simulink model "SF009A_DutyCycThermProtn"  (R2013b)
settings: Solver=FixedStepDiscrete  SolverMode=SingleTasking  StartTime=0.0  StopTime=1  FixedStep=0.1  RelTol=1e-3
values from neighbouring files (symbols this model uses):
  AbsltTThermLimCnt = DataDict.NTC    [SF009A_DutyCycThermProtn_DataDict.m]
  ARCHGLBPRM_100MILLISEC_SEC_F32 = DataDict.Constant    [SF009A_DutyCycThermProtn_DataDict.m]
  CTRLRANDCUTFLT_CNT_U08 = DataDict.Constant    [SF009A_DutyCycThermProtn_DataDict.m]
  CTRLRTFLT_CNT_U08 = DataDict.Constant    [SF009A_DutyCycThermProtn_DataDict.m]
  CUTFLT_CNT_U08 = DataDict.Constant    [SF009A_DutyCycThermProtn_DataDict.m]
  DITHERMLIM_MOTNWTMTR_F32 = DataDict.Constant    [SF009A_DutyCycThermProtn_DataDict.m]
  DutyCycExcddCnt = DataDict.NTC    [SF009A_DutyCycThermProtn_DataDict.m]
  DutyCycThermProtnAbsltCtrlTTblX = DataDict.Calibration    [SF009A_DutyCycThermProtn_DataDict.m]
  DutyCycThermProtnAbsltCtrlTTqTblY = DataDict.Calibration    [SF009A_DutyCycThermProtn_DataDict.m]
  DutyCycThermProtnAbsltCuTTblX = DataDict.Calibration    [SF009A_DutyCycThermProtn_DataDict.m]
  DutyCycThermProtnAbsltCuTTqTblY = DataDict.Calibration    [SF009A_DutyCycThermProtn_DataDict.m]
  DutyCycThermProtnAbsltMotVelBreakPt = DataDict.Calibration    [SF009A_DutyCycThermProtn_DataDict.m]
  DutyCycThermProtnAbsltTTqSlewHiLim = DataDict.Calibration    [SF009A_DutyCycThermProtn_DataDict.m]
  DutyCycThermProtnAbsltTTqSlewLoLim = DataDict.Calibration    [SF009A_DutyCycThermProtn_DataDict.m]
  DutyCycThermProtnCtrlT = DataDict.Calibration    [SF009A_DutyCycThermProtn_DataDict.m]
  DutyCycThermProtnCtrlTSeln = DataDict.Calibration    [SF009A_DutyCycThermProtn_DataDict.m]
  DutyCycThermProtnDutyCycFildThd = DataDict.Calibration    [SF009A_DutyCycThermProtn_DataDict.m]
  DutyCycThermProtnIgnOffCtrlEna = DataDict.Calibration    [SF009A_DutyCycThermProtn_DataDict.m]
  DutyCycThermProtnIgnOffMsgWaitTi = DataDict.Calibration    [SF009A_DutyCycThermProtn_DataDict.m]
  DutyCycThermProtnLstTblValNonStall = DataDict.Calibration    [SF009A_DutyCycThermProtn_DataDict.m]
  DutyCycThermProtnLstTblValStall = DataDict.Calibration    [SF009A_DutyCycThermProtn_DataDict.m]
  DutyCycThermProtnMotPrTSeln = DataDict.Calibration    [SF009A_DutyCycThermProtn_DataDict.m]
  DutyCycThermProtnMplr1NonStallTblY = DataDict.Calibration    [SF009A_DutyCycThermProtn_DataDict.m]
  DutyCycThermProtnMplr1StallTblY = DataDict.Calibration    [SF009A_DutyCycThermProtn_DataDict.m]
  DutyCycThermProtnMplr2NonStallTblY = DataDict.Calibration    [SF009A_DutyCycThermProtn_DataDict.m]
  DutyCycThermProtnMplr2StallTblY = DataDict.Calibration    [SF009A_DutyCycThermProtn_DataDict.m]
  DutyCycThermProtnMplr3NonStallTblY = DataDict.Calibration    [SF009A_DutyCycThermProtn_DataDict.m]
  DutyCycThermProtnMplr3StallTblY = DataDict.Calibration    [SF009A_DutyCycThermProtn_DataDict.m]
  DutyCycThermProtnMplr4NonStallTblY = DataDict.Calibration    [SF009A_DutyCycThermProtn_DataDict.m]
  DutyCycThermProtnMplr4StallTblY = DataDict.Calibration    [SF009A_DutyCycThermProtn_DataDict.m]
  DutyCycThermProtnMplr5NonStallTblY = DataDict.Calibration    [SF009A_DutyCycThermProtn_DataDict.m]
  DutyCycThermProtnMplr5StallTblY = DataDict.Calibration    [SF009A_DutyCycThermProtn_DataDict.m]
  DutyCycThermProtnMplr6NonStallTblY = DataDict.Calibration    [SF009A_DutyCycThermProtn_DataDict.m]
  DutyCycThermProtnMplr6StallTblY = DataDict.Calibration    [SF009A_DutyCycThermProtn_DataDict.m]
  DutyCycThermProtnMplrTblX = DataDict.Calibration    [SF009A_DutyCycThermProtn_DataDict.m]
  DutyCycThermProtnMplrTSeln = DataDict.Calibration    [SF009A_DutyCycThermProtn_DataDict.m]
  DutyCycThermProtnSlowFilTSeln = DataDict.Calibration    [SF009A_DutyCycThermProtn_DataDict.m]
  DutyCycThermProtnThermLimScaFac = DataDict.Calibration    [SF009A_DutyCycThermProtn_DataDict.m]
  DutyCycThermProtnThermLoadLimTblX = DataDict.Calibration    [SF009A_DutyCycThermProtn_DataDict.m]
  DutyCycThermProtnThermLoadLimTblY = DataDict.Calibration    [SF009A_DutyCycThermProtn_DataDict.m]
  DutyCycThermProtnTqCmdSlewDwn = DataDict.Calibration    [SF009A_DutyCycThermProtn_DataDict.m]
  DutyCycThermProtnTqCmdSlewUp = DataDict.Calibration    [SF009A_DutyCycThermProtn_DataDict.m]
  FILVALMIN_ULS_F32 = DataDict.Constant    [SF009A_DutyCycThermProtn_DataDict.m]
  IGNTIOFFTHD_CNT_F32 = DataDict.Constant    [SF009A_DutyCycThermProtn_DataDict.m]
  NODEBSTEP_CNT_U16 = DataDict.Constant    [SF009A_DutyCycThermProtn_DataDict.m]
  ONEPERC_ULS_F32 = DataDict.Constant    [SF009A_DutyCycThermProtn_DataDict.m]
  TAU3_SEC_F32 = DataDict.Constant    [SF009A_DutyCycThermProtn_DataDict.m]
  TAU4_SEC_F32 = DataDict.Constant    [SF009A_DutyCycThermProtn_DataDict.m]
  TAU5_SEC_F32 = DataDict.Constant    [SF009A_DutyCycThermProtn_DataDict.m]
  TAU6_SEC_F32 = DataDict.Constant    [SF009A_DutyCycThermProtn_DataDict.m]
  THERMLOADLIMTBLIDX_ULS_U08 = DataDict.Constant    [SF009A_DutyCycThermProtn_DataDict.m]
undefined symbols (not defined in the file or in its folder): NtcSts1, NvmGetErrSts1
libraries: FixdToFloat x13, Fil x12, NxtrLim x12, simulink x11, NxtrMath x8, FloatToFixd x6, NxtrMax x6, NxtrMin x3, NxtrAbslt x2, NxtrNvM x1
(part 6 of 7)

== system SF009A_DutyCycThermProtn/DutyCycThermProtn/DutyCycThermProtnPer1/LoadLimiting/Multiplier/NonStallCondition ==
  note: Lookup table structure for all tables changed from interpolation to step change for each temperature range.
      | For input values less than the first calibrated X value, the first Y value shall be used, and for input values greater than the largest calibrated X value, the last Y value shall be used.
  note: Non-Stall Condition
  note: Lookup method : Use Input below
  note: Lookup method : Use Input below
  note: Lookup method : Use Input below
  note: Lookup method : Use Input below
  note: Lookup method : Use Input below
  note: Lookup method : Use Input below
  note: The Lookup method used for all the 6 tables below is  "Use Input below" meaning Finds the element in x nearest and below the current input.
      | The corresponding element in y is the output. If there is no element in x below thecurrent input, the block finds the nearest element.
  Mult12Temp : Inport  RequirementInfo={'linktype_rmi_doors' '0000a52a (/E-STEER Core/SubSystem Specifications/Application Functions/SF009A Thermal Duty Cycle Protection)' '#SF009A_224' 'true' 'REQ: SF009A_224' '' } %GIDa_15a3ec26_ae13_4a01_898e_d603e4d6290a
  Mult36TempSlc : Inport  RequirementInfo={'linktype_rmi_doors' '0000a52a (/E-STEER Core/SubSystem Specifications/Application Functions/SF009A Thermal Duty Cycle Protection)' '#SF009A_225' 'true' 'REQ: SF009A_225' '' } %GIDa_709b3fc5_f20d_404f_aaf0_efd71be834f5  Port=2
  Action Port : ActionPort  ActionType=then
  CopyRight2 : Subsystem  Description=|  mask(Copyright Information){none=on}
      | Copyright info block.                                               
      |                                                                     
      | Place copyright information at the top of every subsystem in design.
      mask prompts: none "No parameters"
      mask help: Place copyright information at the top of every subsystem in design.
      mask Display:
      | NxtrConf = 'Nexteer Confidential';
      | 
      | sys = bdroot; %handle for the current model ("system")
      | first = get_param(sys,'Created');
      | first = first(end-3:end);  %year is last four digits
      | 
      | last = get_param(sys,'LastModifiedDate');
      | if isempty(last)
      |     last = datestr(now,'yyyy');
      | else
      |     last = last(end-3:end);
      | end
      | 
      | if strcmp(first,last)
      |     fprintf('%s -- Copyright %s Nexteer',NxtrConf,first)
      | else
      |     fprintf('%s -- %s%s- %s Nexteer',NxtrConf,char(169),first,last)
      | end
  Multiplier 1 Non-Stall Condition Table Lookup : Lookup  RequirementInfo={'linktype_rmi_doors' '0000a52a (/E-STEER Core/SubSystem Specifications/Application Functions/SF009A Thermal Duty Cycle Protection)' '#SF009A_220' 'true' 'REQ: SF009A_220' '' ; 'linktype_rmi_doors' '0000a52a (/E-STEER Core/SubSystem Specifications/Application Functions/SF009A Thermal Duty Cycle Protection)' '#SF009A_222' 'true' 'REQ: SF009A_222' '' } %GIDa_040cbf65_89fb_47d6_bf76_c5ba937961d0  InputValues=DutyCycThermProtnMplrTblX  Table=DutyCycThermProtnMplr1NonStallTblY  LookUpMeth=Use Input Below  OutDataTypeStr=Inherit: Inherit via back propagation
      settings: AttributesFormatString=Output: %<Table>\nInput: %<InputValues>
  Multiplier 2 Non-Stall Condition Table Lookup : Lookup  RequirementInfo={'linktype_rmi_doors' '0000a52a (/E-STEER Core/SubSystem Specifications/Application Functions/SF009A Thermal Duty Cycle Protection)' '#SF009A_220' 'true' 'REQ: SF009A_220' '' ; 'linktype_rmi_doors' '0000a52a (/E-STEER Core/SubSystem Specifications/Application Functions/SF009A Thermal Duty Cycle Protection)' '#SF009A_222' 'true' 'REQ: SF009A_222' '' } %GIDa_8042ba93_215d_4368_8d45_d97009916637  InputValues=DutyCycThermProtnMplrTblX  Table=DutyCycThermProtnMplr2NonStallTblY  LookUpMeth=Use Input Below  OutDataTypeStr=Inherit: Inherit via back propagation
      settings: AttributesFormatString=Output: %<Table>\nInput: %<InputValues>
  Multiplier 3 Non-Stall Condition Table Lookup : Lookup  RequirementInfo={'linktype_rmi_doors' '0000a52a (/E-STEER Core/SubSystem Specifications/Application Functions/SF009A Thermal Duty Cycle Protection)' '#SF009A_220' 'true' 'REQ: SF009A_220' '' ; 'linktype_rmi_doors' '0000a52a (/E-STEER Core/SubSystem Specifications/Application Functions/SF009A Thermal Duty Cycle Protection)' '#SF009A_222' 'true' 'REQ: SF009A_222' '' } %GIDa_e9474d90_bdb6_4f84_bb81_e8f0e810b760  InputValues=DutyCycThermProtnMplrTblX  Table=DutyCycThermProtnMplr3NonStallTblY  LookUpMeth=Use Input Below  OutDataTypeStr=Inherit: Inherit via back propagation
      settings: AttributesFormatString=Output: %<Table>\nInput: %<InputValues>
  Multiplier 4 Non-Stall Condition Table Lookup : Lookup  RequirementInfo={'linktype_rmi_doors' '0000a52a (/E-STEER Core/SubSystem Specifications/Application Functions/SF009A Thermal Duty Cycle Protection)' '#SF009A_220' 'true' 'REQ: SF009A_220' '' ; 'linktype_rmi_doors' '0000a52a (/E-STEER Core/SubSystem Specifications/Application Functions/SF009A Thermal Duty Cycle Protection)' '#SF009A_222' 'true' 'REQ: SF009A_222' '' } %GIDa_5ec721af_8ce5_4ecd_944d_bf56e967375f  InputValues=DutyCycThermProtnMplrTblX  Table=DutyCycThermProtnMplr4NonStallTblY  LookUpMeth=Use Input Below  OutDataTypeStr=Inherit: Inherit via back propagation
      settings: AttributesFormatString=Output: %<Table>\nInput: %<InputValues>
  Multiplier 5 Non-Stall Condition Table Lookup : Lookup  RequirementInfo={'linktype_rmi_doors' '0000a52a (/E-STEER Core/SubSystem Specifications/Application Functions/SF009A Thermal Duty Cycle Protection)' '#SF009A_220' 'true' 'REQ: SF009A_220' '' ; 'linktype_rmi_doors' '0000a52a (/E-STEER Core/SubSystem Specifications/Application Functions/SF009A Thermal Duty Cycle Protection)' '#SF009A_222' 'true' 'REQ: SF009A_222' '' } %GIDa_b08bc230_3876_4054_b57c_d6da79976698  InputValues=DutyCycThermProtnMplrTblX  Table=DutyCycThermProtnMplr5NonStallTblY  LookUpMeth=Use Input Below  OutDataTypeStr=Inherit: Inherit via back propagation
      settings: AttributesFormatString=Output: %<Table>\nInput: %<InputValues>
  Multiplier 6 Non-Stall Condition Table Lookup : Lookup  RequirementInfo={'linktype_rmi_doors' '0000a52a (/E-STEER Core/SubSystem Specifications/Application Functions/SF009A Thermal Duty Cycle Protection)' '#SF009A_220' 'true' 'REQ: SF009A_220' '' ; 'linktype_rmi_doors' '0000a52a (/E-STEER Core/SubSystem Specifications/Application Functions/SF009A Thermal Duty Cycle Protection)' '#SF009A_222' 'true' 'REQ: SF009A_222' '' } %GIDa_31c1cbb5_f611_4930_9dac_12f61a73d29b  InputValues=DutyCycThermProtnMplrTblX  Table=DutyCycThermProtnMplr6NonStallTblY  LookUpMeth=Use Input Below  OutDataTypeStr=Inherit: Inherit via back propagation
      settings: AttributesFormatString=Output: %<Table>\nInput: %<InputValues>
  Mux : Mux  Inputs=6
  Mult : Outport
  wires:
  Multiplier 1 Non-Stall Condition Table Lookup/1 -> Mux/1
  Multiplier 2 Non-Stall Condition Table Lookup/1 -> Mux/2
  Mult36TempSlc/1 -> Multiplier 6 Non-Stall Condition Table Lookup/1, Multiplier 5 Non-Stall Condition Table Lookup/1, Multiplier 3 Non-Stall Condition Table Lookup/1, Multiplier 4 Non-Stall Condition Table Lookup/1
  Multiplier 3 Non-Stall Condition Table Lookup/1 -> Mux/3
  Multiplier 4 Non-Stall Condition Table Lookup/1 -> Mux/4
  Multiplier 5 Non-Stall Condition Table Lookup/1 -> Mux/5
  Multiplier 6 Non-Stall Condition Table Lookup/1 -> Mux/6
  Mult12Temp/1 -> Multiplier 2 Non-Stall Condition Table Lookup/1, Multiplier 1 Non-Stall Condition Table Lookup/1
  Mux/1 -> Mult/1

== system SF009A_DutyCycThermProtn/DutyCycThermProtn/DutyCycThermProtnPer1/LoadLimiting/Multiplier/SlowFilTSeln_Mult12Temp ==
  Mult12Temp : Inport
  Action Port : ActionPort  ActionType=then
  CopyRight2 : Subsystem  Description=|  mask(Copyright Information){none=on}
      | Copyright info block.                                               
      |                                                                     
      | Place copyright information at the top of every subsystem in design.
      mask prompts: none "No parameters"
      mask help: Place copyright information at the top of every subsystem in design.
      mask Display:
      | NxtrConf = 'Nexteer Confidential';
      | 
      | sys = bdroot; %handle for the current model ("system")
      | first = get_param(sys,'Created');
      | first = first(end-3:end);  %year is last four digits
      | 
      | last = get_param(sys,'LastModifiedDate');
      | if isempty(last)
      |     last = datestr(now,'yyyy');
      | else
      |     last = last(end-3:end);
      | end
      | 
      | if strcmp(first,last)
      |     fprintf('%s -- Copyright %s Nexteer',NxtrConf,first)
      | else
      |     fprintf('%s -- %s%s- %s Nexteer',NxtrConf,char(169),first,last)
      | end
  Mult36TempSlc : Outport
  wires:
  Mult12Temp/1 -> Mult36TempSlc/1

== system SF009A_DutyCycThermProtn/DutyCycThermProtn/DutyCycThermProtnPer1/LoadLimiting/Multiplier/SlowFilTSeln_Mult36Temp ==
  Mult36Temp : Inport
  Action Port : ActionPort  ActionType=else
  CopyRight2 : Subsystem  Description=|  mask(Copyright Information){none=on}
      | Copyright info block.                                               
      |                                                                     
      | Place copyright information at the top of every subsystem in design.
      mask prompts: none "No parameters"
      mask help: Place copyright information at the top of every subsystem in design.
      mask Display:
      | NxtrConf = 'Nexteer Confidential';
      | 
      | sys = bdroot; %handle for the current model ("system")
      | first = get_param(sys,'Created');
      | first = first(end-3:end);  %year is last four digits
      | 
      | last = get_param(sys,'LastModifiedDate');
      | if isempty(last)
      |     last = datestr(now,'yyyy');
      | else
      |     last = last(end-3:end);
      | end
      | 
      | if strcmp(first,last)
      |     fprintf('%s -- Copyright %s Nexteer',NxtrConf,first)
      | else
      |     fprintf('%s -- %s%s- %s Nexteer',NxtrConf,char(169),first,last)
      | end
  Mult36TempSlc : Outport
  wires:
  Mult36Temp/1 -> Mult36TempSlc/1

== system SF009A_DutyCycThermProtn/DutyCycThermProtn/DutyCycThermProtnPer1/LoadLimiting/Multiplier/StallCondition ==
  note: Lookup table structure for all tables changed from interpolation to step change for each temperature range.
      | For input values less than the first calibrated X value, the first Y value shall be used, and for input values greater than the largest calibrated X value, the last Y value shall be used.
  note: Stall Condition
  note: The Lookup method used for all the 6 tables below is  "Use Input below" meaning Finds the element in x nearest and below the current input.
      | The corresponding element in y is the output. If there is no element in x below thecurrent input, the block finds the nearest element.
  note: Lookup method : Use Input below
  note: Lookup method : Use Input below
  note: Lookup method : Use Input below
  note: Lookup method : Use Input below
  note: Lookup method : Use Input below
  note: Lookup method : Use Input below
  Mult12Temp : Inport  RequirementInfo={'linktype_rmi_doors' '0000a52a (/E-STEER Core/SubSystem Specifications/Application Functions/SF009A Thermal Duty Cycle Protection)' '#SF009A_224' 'true' 'REQ: SF009A_224' '' } %GIDa_9e736f64_5371_48c6_b29d_98d7a04e2700
  Mult36TempSlc : Inport  RequirementInfo={'linktype_rmi_doors' '0000a52a (/E-STEER Core/SubSystem Specifications/Application Functions/SF009A Thermal Duty Cycle Protection)' '#SF009A_225' 'true' 'REQ: SF009A_225' '' } %GIDa_553df6a3_e81e_4199_bb36_62f8d0306279  Port=2
  Action Port : ActionPort  ActionType=else
  CopyRight2 : Subsystem  Description=|  mask(Copyright Information){none=on}
      | Copyright info block.                                               
      |                                                                     
      | Place copyright information at the top of every subsystem in design.
      mask prompts: none "No parameters"
      mask help: Place copyright information at the top of every subsystem in design.
      mask Display:
      | NxtrConf = 'Nexteer Confidential';
      | 
      | sys = bdroot; %handle for the current model ("system")
      | first = get_param(sys,'Created');
      | first = first(end-3:end);  %year is last four digits
      | 
      | last = get_param(sys,'LastModifiedDate');
      | if isempty(last)
      |     last = datestr(now,'yyyy');
      | else
      |     last = last(end-3:end);
      | end
      | 
      | if strcmp(first,last)
      |     fprintf('%s -- Copyright %s Nexteer',NxtrConf,first)
      | else
      |     fprintf('%s -- %s%s- %s Nexteer',NxtrConf,char(169),first,last)
      | end
  Multiplier 1 Stall Condition Table Lookup : Lookup  RequirementInfo={'linktype_rmi_doors' '0000a52a (/E-STEER Core/SubSystem Specifications/Application Functions/SF009A Thermal Duty Cycle Protection)' '#SF009A_221' 'true' 'REQ: SF009A_221' '' ; 'linktype_rmi_doors' '0000a52a (/E-STEER Core/SubSystem Specifications/Application Functions/SF009A Thermal Duty Cycle Protection)' '#SF009A_222' 'true' 'REQ: SF009A_222' '' } %GIDa_9fd8bddf_55f4_40c2_9de1_5afa276fb2ae  InputValues=DutyCycThermProtnMplrTblX  Table=DutyCycThermProtnMplr1StallTblY  LookUpMeth=Use Input Below  OutDataTypeStr=Inherit: Inherit via back propagation
      settings: AttributesFormatString=Output: %<Table>\nInput: %<InputValues>
  Multiplier 2 Stall Condition Table Lookup : Lookup  RequirementInfo={'linktype_rmi_doors' '0000a52a (/E-STEER Core/SubSystem Specifications/Application Functions/SF009A Thermal Duty Cycle Protection)' '#SF009A_221' 'true' 'REQ: SF009A_221' '' ; 'linktype_rmi_doors' '0000a52a (/E-STEER Core/SubSystem Specifications/Application Functions/SF009A Thermal Duty Cycle Protection)' '#SF009A_222' 'true' 'REQ: SF009A_222' '' } %GIDa_d13a61f9_bc55_4f9c_9c82_b67ebcc5711f  InputValues=DutyCycThermProtnMplrTblX  Table=DutyCycThermProtnMplr2StallTblY  LookUpMeth=Use Input Below  OutDataTypeStr=Inherit: Inherit via back propagation
      settings: AttributesFormatString=Output: %<Table>\nInput: %<InputValues>
  Multiplier 3 Stall Condition Table Lookup : Lookup  RequirementInfo={'linktype_rmi_doors' '0000a52a (/E-STEER Core/SubSystem Specifications/Application Functions/SF009A Thermal Duty Cycle Protection)' '#SF009A_221' 'true' 'REQ: SF009A_221' '' ; 'linktype_rmi_doors' '0000a52a (/E-STEER Core/SubSystem Specifications/Application Functions/SF009A Thermal Duty Cycle Protection)' '#SF009A_222' 'true' 'REQ: SF009A_222' '' } %GIDa_e78f92bd_c818_4426_875e_d4129946569a  InputValues=DutyCycThermProtnMplrTblX  Table=DutyCycThermProtnMplr3StallTblY  LookUpMeth=Use Input Below  OutDataTypeStr=Inherit: Inherit via back propagation
      settings: AttributesFormatString=Output: %<Table>\nInput: %<InputValues>
  Multiplier 4 Stall Condition Table Lookup : Lookup  RequirementInfo={'linktype_rmi_doors' '0000a52a (/E-STEER Core/SubSystem Specifications/Application Functions/SF009A Thermal Duty Cycle Protection)' '#SF009A_221' 'true' 'REQ: SF009A_221' '' ; 'linktype_rmi_doors' '0000a52a (/E-STEER Core/SubSystem Specifications/Application Functions/SF009A Thermal Duty Cycle Protection)' '#SF009A_222' 'true' 'REQ: SF009A_222' '' } %GIDa_54fd5508_1ae5_4eef_8010_89a382576046  InputValues=DutyCycThermProtnMplrTblX  Table=DutyCycThermProtnMplr4StallTblY  LookUpMeth=Use Input Below  OutDataTypeStr=Inherit: Inherit via back propagation
      settings: AttributesFormatString=Output: %<Table>\nInput: %<InputValues>
  Multiplier 5 Stall Condition Table Lookup : Lookup  RequirementInfo={'linktype_rmi_doors' '0000a52a (/E-STEER Core/SubSystem Specifications/Application Functions/SF009A Thermal Duty Cycle Protection)' '#SF009A_221' 'true' 'REQ: SF009A_221' '' ; 'linktype_rmi_doors' '0000a52a (/E-STEER Core/SubSystem Specifications/Application Functions/SF009A Thermal Duty Cycle Protection)' '#SF009A_222' 'true' 'REQ: SF009A_222' '' } %GIDa_564254f9_1620_4814_afcf_4fcd885d6474  InputValues=DutyCycThermProtnMplrTblX  Table=DutyCycThermProtnMplr5StallTblY  LookUpMeth=Use Input Below  OutDataTypeStr=Inherit: Inherit via back propagation
      settings: AttributesFormatString=Output: %<Table>\nInput: %<InputValues>
  Multiplier 6 Stall Condition Table Lookup : Lookup  RequirementInfo={'linktype_rmi_doors' '0000a52a (/E-STEER Core/SubSystem Specifications/Application Functions/SF009A Thermal Duty Cycle Protection)' '#SF009A_221' 'true' 'REQ: SF009A_221' '' ; 'linktype_rmi_doors' '0000a52a (/E-STEER Core/SubSystem Specifications/Application Functions/SF009A Thermal Duty Cycle Protection)' '#SF009A_222' 'true' 'REQ: SF009A_222' '' } %GIDa_199596d5_92a0_4d88_bfbd_ade09bff1f42  InputValues=DutyCycThermProtnMplrTblX  Table=DutyCycThermProtnMplr6StallTblY  LookUpMeth=Use Input Below  OutDataTypeStr=Inherit: Inherit via back propagation
      settings: AttributesFormatString=Output: %<Table>\nInput: %<InputValues>
  Mux : Mux  Inputs=6
  Mult : Outport
  wires:
  Multiplier 1 Stall Condition Table Lookup/1 -> Mux/1
  Multiplier 4 Stall Condition Table Lookup/1 -> Mux/4
  Mult12Temp/1 -> Multiplier 1 Stall Condition Table Lookup/1, Multiplier 2 Stall Condition Table Lookup/1
  Mult36TempSlc/1 -> Multiplier 3 Stall Condition Table Lookup/1, Multiplier 4 Stall Condition Table Lookup/1, Multiplier 5 Stall Condition Table Lookup/1, Multiplier 6 Stall Condition Table Lookup/1
  Multiplier 2 Stall Condition Table Lookup/1 -> Mux/2
  Multiplier 5 Stall Condition Table Lookup/1 -> Mux/5
  Multiplier 6 Stall Condition Table Lookup/1 -> Mux/6
  Multiplier 3 Stall Condition Table Lookup/1 -> Mux/3
  Mux/1 -> Mult/1

== system SF009A_DutyCycThermProtn/DutyCycThermProtn/DutyCycThermProtnPer1/LoadLimiting/PowerOffTasks/CopyRight2 ==

== system SF009A_DutyCycThermProtn/DutyCycThermProtn/DutyCycThermProtnPer1/LoadLimiting/ThermalLoadLimit/CopyRight2 ==

== system SF009A_DutyCycThermProtn/DutyCycThermProtn/DutyCycThermProtnPer1/LoadLimiting/ThermalLoadLimit/DutyCycleLevel_LstTblValNonStall ==
  Action Port : ActionPort  ActionType=then
  Constant : Constant  RequirementInfo={'linktype_rmi_doors' '0000a52a (/E-STEER Core/SubSystem Specifications/Application Functions/SF009A Thermal Duty Cycle Protection)' '#SF009A_237' 'true' 'REQ: SF009A_237' '' } %GIDa_2bdb37b2_90de_4932_bdc4_6093f9667a46  Value=DutyCycThermProtnLstTblValNonStall
  CopyRight2 : Subsystem  Description=|  mask(Copyright Information){none=on}
      | Copyright info block.                                               
      |                                                                     
      | Place copyright information at the top of every subsystem in design.
      mask prompts: none "No parameters"
      mask help: Place copyright information at the top of every subsystem in design.
      mask Display:
      | NxtrConf = 'Nexteer Confidential';
      | 
      | sys = bdroot; %handle for the current model ("system")
      | first = get_param(sys,'Created');
      | first = first(end-3:end);  %year is last four digits
      | 
      | last = get_param(sys,'LastModifiedDate');
      | if isempty(last)
      |     last = datestr(now,'yyyy');
      | else
      |     last = last(end-3:end);
      | end
      | 
      | if strcmp(first,last)
      |     fprintf('%s -- Copyright %s Nexteer',NxtrConf,first)
      | else
      |     fprintf('%s -- %s%s- %s Nexteer',NxtrConf,char(169),first,last)
      | end
  DutyCycleLevel : Outport
  wires:
  Constant/1 -> DutyCycleLevel/1

== system SF009A_DutyCycThermProtn/DutyCycThermProtn/DutyCycThermProtnPer1/LoadLimiting/ThermalLoadLimit/DutyCycleLevel_LstTblValStall ==
  Action Port : ActionPort  ActionType=else
  CopyRight2 : Subsystem  Description=|  mask(Copyright Information){none=on}
      | Copyright info block.                                               
      |                                                                     
      | Place copyright information at the top of every subsystem in design.
      mask prompts: none "No parameters"
      mask help: Place copyright information at the top of every subsystem in design.
      mask Display:
      | NxtrConf = 'Nexteer Confidential';
      | 
      | sys = bdroot; %handle for the current model ("system")
      | first = get_param(sys,'Created');
      | first = first(end-3:end);  %year is last four digits
      | 
      | last = get_param(sys,'LastModifiedDate');
      | if isempty(last)
      |     last = datestr(now,'yyyy');
      | else
      |     last = last(end-3:end);
      | end
      | 
      | if strcmp(first,last)
      |     fprintf('%s -- Copyright %s Nexteer',NxtrConf,first)
      | else
      |     fprintf('%s -- %s%s- %s Nexteer',NxtrConf,char(169),first,last)
      | end
  Thermal Load (Torque Command) Limit Table2 : Constant  RequirementInfo={'linktype_rmi_doors' '0000a52a (/E-STEER Core/SubSystem Specifications/Application Functions/SF009A Thermal Duty Cycle Protection)' '#SF009A_238' 'true' 'REQ: SF009A_238' '' } %GIDa_b4fdb058_87f9_43b9_9a91_a70718fca0fe  Value=DutyCycThermProtnLstTblValStall
  DutyCycleLevel : Outport
  wires:
  Thermal Load (Torque Command) Limit Table2/1 -> DutyCycleLevel/1

== system SF009A_DutyCycThermProtn/DutyCycThermProtn/DutyCycThermProtnPer1/TemperatureSelection/MplrTSelnDisabled/CopyRight2 ==

== system SF009A_DutyCycThermProtn/DutyCycThermProtn/DutyCycThermProtnPer1/TemperatureSelection/MplrTSelnEnabled/CopyRight2 ==

== system SF009A_DutyCycThermProtn/DutyCycThermProtn/DutyCycThermProtnPer1/TemperatureSelection/Mult12T_DiagcStsLimdTPrfmncDisabled/CopyRight2 ==

== system SF009A_DutyCycThermProtn/DutyCycThermProtn/DutyCycThermProtnPer1/TemperatureSelection/Mult12T_DiagcStsLimdTPrfmncDisabled/CtrlTSelnDisabled ==
  MotFetT : Inport
  Action Port : ActionPort  ActionType=else
  CopyRight2 : Subsystem  Description=|  mask(Copyright Information){none=on}
      | Copyright info block.                                               
      |                                                                     
      | Place copyright information at the top of every subsystem in design.
      mask prompts: none "No parameters"
      mask help: Place copyright information at the top of every subsystem in design.
      mask Display:
      | NxtrConf = 'Nexteer Confidential';
      | 
      | sys = bdroot; %handle for the current model ("system")
      | first = get_param(sys,'Created');
      | first = first(end-3:end);  %year is last four digits
      | 
      | last = get_param(sys,'LastModifiedDate');
      | if isempty(last)
      |     last = datestr(now,'yyyy');
      | else
      |     last = last(end-3:end);
      | end
      | 
      | if strcmp(first,last)
      |     fprintf('%s -- Copyright %s Nexteer',NxtrConf,first)
      | else
      |     fprintf('%s -- %s%s- %s Nexteer',NxtrConf,char(169),first,last)
      | end
  Mult12 : Outport
  wires:
  MotFetT/1 -> Mult12/1

== system SF009A_DutyCycThermProtn/DutyCycThermProtn/DutyCycThermProtnPer1/TemperatureSelection/Mult12T_DiagcStsLimdTPrfmncDisabled/CtrlTSelnEnabled ==
  EcuTFild : Inport
  Action Port : ActionPort  ActionType=then
  CopyRight2 : Subsystem  Description=|  mask(Copyright Information){none=on}
      | Copyright info block.                                               
      |                                                                     
      | Place copyright information at the top of every subsystem in design.
      mask prompts: none "No parameters"
      mask help: Place copyright information at the top of every subsystem in design.
      mask Display:
      | NxtrConf = 'Nexteer Confidential';
      | 
      | sys = bdroot; %handle for the current model ("system")
      | first = get_param(sys,'Created');
      | first = first(end-3:end);  %year is last four digits
      | 
      | last = get_param(sys,'LastModifiedDate');
      | if isempty(last)
      |     last = datestr(now,'yyyy');
      | else
      |     last = last(end-3:end);
      | end
      | 
      | if strcmp(first,last)
      |     fprintf('%s -- Copyright %s Nexteer',NxtrConf,first)
      | else
      |     fprintf('%s -- %s%s- %s Nexteer',NxtrConf,char(169),first,last)
      | end
  Mult12 : Outport
  wires:
  EcuTFild/1 -> Mult12/1

== system SF009A_DutyCycThermProtn/DutyCycThermProtn/DutyCycThermProtnPer1/TemperatureSelection/Mult12T_DiagcStsLimdTPrfmncEnabled/CopyRight2 ==

== system SF009A_DutyCycThermProtn/DutyCycThermProtn/DutyCycThermProtnPer1/TemperatureSelection/Mult36T_DiagcStsLimdTPrfmncDisabled/CopyRight2 ==

== system SF009A_DutyCycThermProtn/DutyCycThermProtn/DutyCycThermProtnPer1/TemperatureSelection/Mult36T_DiagcStsLimdTPrfmncDisabled/MotPrTSelnDisabled ==
  MotWidgT : Inport
  Action Port : ActionPort  ActionType=else
  CopyRight2 : Subsystem  Description=|  mask(Copyright Information){none=on}
      | Copyright info block.                                               
      |                                                                     
      | Place copyright information at the top of every subsystem in design.
      mask prompts: none "No parameters"
      mask help: Place copyright information at the top of every subsystem in design.
      mask Display:
      | NxtrConf = 'Nexteer Confidential';
      | 
      | sys = bdroot; %handle for the current model ("system")
      | first = get_param(sys,'Created');
      | first = first(end-3:end);  %year is last four digits
      | 
      | last = get_param(sys,'LastModifiedDate');
      | if isempty(last)
      |     last = datestr(now,'yyyy');
      | else
      |     last = last(end-3:end);
      | end
      | 
      | if strcmp(first,last)
      |     fprintf('%s -- Copyright %s Nexteer',NxtrConf,first)
      | else
      |     fprintf('%s -- %s%s- %s Nexteer',NxtrConf,char(169),first,last)
      | end
  Mult36 : Outport
  wires:
  MotWidgT/1 -> Mult36/1

== system SF009A_DutyCycThermProtn/DutyCycThermProtn/DutyCycThermProtnPer1/TemperatureSelection/Mult36T_DiagcStsLimdTPrfmncDisabled/MotPrTSelnEnabled ==
  MotMagT : Inport
  Action Port : ActionPort  ActionType=then
  CopyRight2 : Subsystem  Description=|  mask(Copyright Information){none=on}
      | Copyright info block.                                               
      |                                                                     
      | Place copyright information at the top of every subsystem in design.
      mask prompts: none "No parameters"
      mask help: Place copyright information at the top of every subsystem in design.
      mask Display:
      | NxtrConf = 'Nexteer Confidential';
      | 
      | sys = bdroot; %handle for the current model ("system")
      | first = get_param(sys,'Created');
      | first = first(end-3:end);  %year is last four digits
      | 
      | last = get_param(sys,'LastModifiedDate');
      | if isempty(last)
      |     last = datestr(now,'yyyy');
      | else
      |     last = last(end-3:end);
      | end
      | 
      | if strcmp(first,last)
      |     fprintf('%s -- Copyright %s Nexteer',NxtrConf,first)
      | else
      |     fprintf('%s -- %s%s- %s Nexteer',NxtrConf,char(169),first,last)
      | end
  Mult36 : Outport
  wires:
  MotMagT/1 -> Mult36/1

== system SF009A_DutyCycThermProtn/DutyCycThermProtn/DutyCycThermProtnPer1/TemperatureSelection/Mult36T_DiagcStsLimdTPrfmncEnabled/CopyRight2 ==

== system SF009A_DutyCycThermProtn/DutyCycThermProtn/DutyCycThermProtnPer1/TempratureLimiting/SetCtrlrAndCuTFltNtc/CopyRight2 ==

== system SF009A_DutyCycThermProtn/DutyCycThermProtn/DutyCycThermProtnPer1/TempratureLimiting/SetCtrlrTFltNtc/CopyRight2 ==

== system SF009A_DutyCycThermProtn/DutyCycThermProtn/DutyCycThermProtnPer1/TempratureLimiting/SetCuTFltNtc/CopyRight2 ==

== system SF009A_DutyCycThermProtn/DutyCycThermProtn/DutyCycThermProtnPer1/TempratureLimiting/SetNtc/CopyRight2 ==

== system SF009A_DutyCycThermProtn/DutyCycThermProtn/DutyCycThermProtnPer1/TempratureLimiting/SetNtc/SetNtcSts ==
  note: Note:
      |
      | - "ISO Fault Debounce Design" Simulink block intent to use here for Simulation purpose only. Do not Code this block
  NtcNr : Inport
  NtcStInfo : Inport  Port=2
  NtcSts : Inport  Port=3
  DebStep : Inport  Port=4
  Copyright1 : Subsystem  Description=|  RequirementInfo={} %GIDa_eb45801b_6e45_4d0e_85d0_27f2c30c63b6  mask(Copyright Information){none=on}
      | Copyright info block.                                               
      |                                                                     
      | Place copyright information at the top of every subsystem in design.
      mask prompts: none "No parameters"
      mask help: Place copyright information at the top of every subsystem in design.
      mask Display:
      | NxtrConf = 'Nexteer Confidential';
      | 
      | sys = bdroot; %handle for the current model ("system")
      | first = get_param(sys,'Created');
      | if(isempty(first))
      |     first = datestr(now,'yyyy');
      | else
      |     first = first(end-3:end);  %year is last four digits
      | end
      | 
      | last = get_param(sys,'LastModifiedDate');
      | if isempty(last)
      |     last = datestr(now,'yyyy');
      | else
      |     last = last(end-3:end);
      | end
      | 
      | if strcmp(first,last)
      |     fprintf('%s\nCopyright  %s Nexteer',NxtrConf,first);
      | else
      |     fprintf('%s\n%s%s-%s Nexteer',NxtrConf,char(169),first,last);
      | end
  Data Store Write : DataStoreWrite  DataStoreName=AbsltTThermLimCntQlfr
  Data Store Write2 : DataStoreWrite  DataStoreName=AbsltTThermLimCntStInfo
  Data Store Write3 : DataStoreWrite  DataStoreName=AbsltTThermLimCntStsVal
  Data Type Conversion : DataTypeConversion  OutDataTypeStr=Enum: SigQlfr1
  Ground : Ground
  ISO Fault Debounce Design : Stateflow chart  TreatAsAtomicUnit=on
      settings: AttributesFormatString=|
      | Simulation Purpose Only.
      | Do Not Code this block
      | Diagnostic Manager Owns this requirement
  Terminator : Terminator
  Terminator1 : Terminator
  wires:
  NtcNr/1 -> Terminator/1
  NtcStInfo/1 -> Data Store Write2/1, Terminator1/1
  DebStep/1 -> ISO Fault Debounce Design/2(DebStep)
  Ground/1 -> ISO Fault Debounce Design/3(SvcClr)
  NtcSts/1 -> Data Store Write3/1, ISO Fault Debounce Design/1(NtcSts)
  ISO Fault Debounce Design/1(Qualifier) -> Data Type Conversion/1
  Data Type Conversion/1 -> Data Store Write/1

== system SF009A_DutyCycThermProtn/DutyCycThermProtn/DutyCycThermProtnPer1/TempratureLimiting/SetPassdNtc/CopyRight2 ==

== system SF009A_DutyCycThermProtn/DutyCycThermProtn/DutyCycThermProtnPer1/ThermalLimitStatus/DutyCycThermProtnDisabled/CopyRight2 ==

== system SF009A_DutyCycThermProtn/DutyCycThermProtn/DutyCycThermProtnPer1/ThermalLimitStatus/DutyCycThermProtnEnabled /CopyRight2 ==

== system SF009A_DutyCycThermProtn/DutyCycThermProtn/DutyCycThermProtnPer1/ThermalLimitStatus/MaxoutLimiting/CopyRight2 ==

== system SF009A_DutyCycThermProtn/DutyCycThermProtn/DutyCycThermProtnPer1/ThermalLimitStatus/MaxoutLimiting/SetNtcFail ==
  NtcNr : Inport
  NtcStInfo : Inport  Port=2
  NtcSts : Inport  Port=3
  DebStep : Inport  Port=4
  Action Port : ActionPort  ActionType=else
  Copyright1 : Subsystem  Description=|  RequirementInfo={} %GIDa_c870bdf9_6ce0_40fe_bc65_b64ff8059a8b  mask(Copyright Information){none=on}
      | Copyright info block.                                               
      |                                                                     
      | Place copyright information at the top of every subsystem in design.
      mask prompts: none "No parameters"
      mask help: Place copyright information at the top of every subsystem in design.
      mask Display:
      | NxtrConf = 'Nexteer Confidential';
      | 
      | sys = bdroot; %handle for the current model ("system")
      | first = get_param(sys,'Created');
      | if(isempty(first))
      |     first = datestr(now,'yyyy');
      | else
      |     first = first(end-3:end);  %year is last four digits
      | end
      | 
      | last = get_param(sys,'LastModifiedDate');
      | if isempty(last)
      |     last = datestr(now,'yyyy');
      | else
      |     last = last(end-3:end);
      | end
      | 
      | if strcmp(first,last)
      |     fprintf('%s\nCopyright  %s Nexteer',NxtrConf,first);
      | else
      |     fprintf('%s\n%s%s-%s Nexteer',NxtrConf,char(169),first,last);
      | end
  SetNtcSts : Subsystem  RequirementInfo={} %GIDa_a9f1dd79_07fa_4e28_8f86_fa6802a724f4
  wires:
  DebStep/1 -> SetNtcSts/4(DebStep)
  NtcSts/1 -> SetNtcSts/3(NtcSts)
  NtcStInfo/1 -> SetNtcSts/2(NtcStInfo)
  NtcNr/1 -> SetNtcSts/1(NtcNr)

== system SF009A_DutyCycThermProtn/DutyCycThermProtn/DutyCycThermProtnPer1/ThermalLimitStatus/MaxoutLimiting/SetNtcPass ==
  NtcNr : Inport
  NtcStInfo : Inport  Port=2
  NtcSts : Inport  Port=3
  DebStep : Inport  Port=4
  Action Port : ActionPort  ActionType=then
  Copyright1 : Subsystem  Description=|  RequirementInfo={} %GIDa_0ced068a_7ed3_40c3_85e7_3b3aa7f7abba  mask(Copyright Information){none=on}
      | Copyright info block.                                               
      |                                                                     
      | Place copyright information at the top of every subsystem in design.
      mask prompts: none "No parameters"
      mask help: Place copyright information at the top of every subsystem in design.
      mask Display:
      | NxtrConf = 'Nexteer Confidential';
      | 
      | sys = bdroot; %handle for the current model ("system")
      | first = get_param(sys,'Created');
      | if(isempty(first))
      |     first = datestr(now,'yyyy');
      | else
      |     first = first(end-3:end);  %year is last four digits
      | end
      | 
      | last = get_param(sys,'LastModifiedDate');
      | if isempty(last)
      |     last = datestr(now,'yyyy');
      | else
      |     last = last(end-3:end);
      | end
      | 
      | if strcmp(first,last)
      |     fprintf('%s\nCopyright  %s Nexteer',NxtrConf,first);
      | else
      |     fprintf('%s\n%s%s-%s Nexteer',NxtrConf,char(169),first,last);
      | end
  SetNtcSts : Subsystem  RequirementInfo={} %GIDa_a1e7f663_1c82_4c2b_bb27_c1170dac376e
  wires:
  NtcNr/1 -> SetNtcSts/1(NtcNr)
  NtcStInfo/1 -> SetNtcSts/2(NtcStInfo)
  NtcSts/1 -> SetNtcSts/3(NtcSts)
  DebStep/1 -> SetNtcSts/4(DebStep)

== system SF009A_DutyCycThermProtn/DutyCycThermProtn/DutyCycThermProtnPer1/TherrmalLimitScaling/ThermDutyCycLoadDptDisabled /CopyRight2 ==

== system SF009A_DutyCycThermProtn/DutyCycThermProtn/DutyCycThermProtnPer1/TherrmalLimitScaling/ThermDutyCycLoadDptEnabled/CopyRight2 ==

== system SF009A_DutyCycThermProtn/DutyCycThermProtn/DutyCycThermProtnPer1/TherrmalLimitScaling/ThermLim_DutyCycThermProtnDisabled1/CopyRight2 ==

== system SF009A_DutyCycThermProtn/DutyCycThermProtn/DutyCycThermProtnPer1/TherrmalLimitScaling/ThermLim_DutyCycThermProtnDisabled2/CopyRight2 ==

== system SF009A_DutyCycThermProtn/DutyCycThermProtn/DutyCycThermProtnPer1/TherrmalLimitScaling/ThermLim_DutyCycThermProtnEnabled1/CopyRight2 ==

== system SF009A_DutyCycThermProtn/DutyCycThermProtn/DutyCycThermProtnPer1/TherrmalLimitScaling/ThermLim_DutyCycThermProtnEnabled2/CopyRight2 ==

== system SF009A_DutyCycThermProtn/DutyCycThermProtn/DutyCycThermProtnInit1/PowerOnTasks/InputIgnOffTime/Filt3ExpDecay/CopyRight2 ==

== system SF009A_DutyCycThermProtn/DutyCycThermProtn/DutyCycThermProtnInit1/PowerOnTasks/InputIgnOffTime/Filt4ExpDecay/CopyRight2 ==

== system SF009A_DutyCycThermProtn/DutyCycThermProtn/DutyCycThermProtnInit1/PowerOnTasks/InputIgnOffTime/Filt5ExpDecay/CopyRight2 ==

== system SF009A_DutyCycThermProtn/DutyCycThermProtn/DutyCycThermProtnInit1/PowerOnTasks/InputIgnOffTime/Filt6ExpDecay/CopyRight2 ==

== system SF009A_DutyCycThermProtn/DutyCycThermProtn/DutyCycThermProtnPer1/FiltSVReinit/VehTiVldEnabled/Filt3ExpDecay/CopyRight2 ==

== system SF009A_DutyCycThermProtn/DutyCycThermProtn/DutyCycThermProtnPer1/FiltSVReinit/VehTiVldEnabled/Filt4ExpDecay/CopyRight2 ==

== system SF009A_DutyCycThermProtn/DutyCycThermProtn/DutyCycThermProtnPer1/FiltSVReinit/VehTiVldEnabled/Filt5ExpDecay/CopyRight2 ==

== system SF009A_DutyCycThermProtn/DutyCycThermProtn/DutyCycThermProtnPer1/FiltSVReinit/VehTiVldEnabled/Filt6ExpDecay/CopyRight2 ==

== system SF009A_DutyCycThermProtn/DutyCycThermProtn/DutyCycThermProtnPer1/LoadLimiting/FilterPercMax/DutyCycLevel_DutyCycThermProtnDisabled/CopyRight2 ==

== system SF009A_DutyCycThermProtn/DutyCycThermProtn/DutyCycThermProtnPer1/LoadLimiting/FilterPercMax/DutyCycLevel_DutyCycThermProtnEnabled/CopyRight2 ==

== system SF009A_DutyCycThermProtn/DutyCycThermProtn/DutyCycThermProtnPer1/LoadLimiting/Multiplier/NonStallCondition/CopyRight2 ==

== system SF009A_DutyCycThermProtn/DutyCycThermProtn/DutyCycThermProtnPer1/LoadLimiting/Multiplier/SlowFilTSeln_Mult12Temp/CopyRight2 ==

== system SF009A_DutyCycThermProtn/DutyCycThermProtn/DutyCycThermProtnPer1/LoadLimiting/Multiplier/SlowFilTSeln_Mult36Temp/CopyRight2 ==

== system SF009A_DutyCycThermProtn/DutyCycThermProtn/DutyCycThermProtnPer1/LoadLimiting/Multiplier/StallCondition/CopyRight2 ==

== system SF009A_DutyCycThermProtn/DutyCycThermProtn/DutyCycThermProtnPer1/LoadLimiting/ThermalLoadLimit/DutyCycleLevel_LstTblValNonStall/CopyRight2 ==

== system SF009A_DutyCycThermProtn/DutyCycThermProtn/DutyCycThermProtnPer1/LoadLimiting/ThermalLoadLimit/DutyCycleLevel_LstTblValStall/CopyRight2 ==

== system SF009A_DutyCycThermProtn/DutyCycThermProtn/DutyCycThermProtnPer1/TemperatureSelection/Mult12T_DiagcStsLimdTPrfmncDisabled/CtrlTSelnDisabled/CopyRight2 ==

== system SF009A_DutyCycThermProtn/DutyCycThermProtn/DutyCycThermProtnPer1/TemperatureSelection/Mult12T_DiagcStsLimdTPrfmncDisabled/CtrlTSelnEnabled/CopyRight2 ==

== system SF009A_DutyCycThermProtn/DutyCycThermProtn/DutyCycThermProtnPer1/TemperatureSelection/Mult36T_DiagcStsLimdTPrfmncDisabled/MotPrTSelnDisabled/CopyRight2 ==

== system SF009A_DutyCycThermProtn/DutyCycThermProtn/DutyCycThermProtnPer1/TemperatureSelection/Mult36T_DiagcStsLimdTPrfmncDisabled/MotPrTSelnEnabled/CopyRight2 ==

== system SF009A_DutyCycThermProtn/DutyCycThermProtn/DutyCycThermProtnPer1/TempratureLimiting/SetNtc/SetNtcSts/Copyright1 ==

== system SF009A_DutyCycThermProtn/DutyCycThermProtn/DutyCycThermProtnPer1/ThermalLimitStatus/MaxoutLimiting/SetNtcFail/Copyright1 ==

== system SF009A_DutyCycThermProtn/DutyCycThermProtn/DutyCycThermProtnPer1/ThermalLimitStatus/MaxoutLimiting/SetNtcFail/SetNtcSts ==
  note: Note:
      |
      | - "ISO Fault Debounce Design" Simulink block intent to use here for Simulation purpose only. Do not Code this block
  NtcNr : Inport
  NtcStInfo : Inport  Port=2
  NtcSts : Inport  Port=3
  DebStep : Inport  Port=4
  Copyright1 : Subsystem  Description=|  RequirementInfo={} %GIDa_da6c99a2_667b_4a6d_9355_eed1021c382c  mask(Copyright Information){none=on}
      | Copyright info block.                                               
      |                                                                     
      | Place copyright information at the top of every subsystem in design.
      mask prompts: none "No parameters"
      mask help: Place copyright information at the top of every subsystem in design.
      mask Display:
      | NxtrConf = 'Nexteer Confidential';
      | 
      | sys = bdroot; %handle for the current model ("system")
      | first = get_param(sys,'Created');
      | if(isempty(first))
      |     first = datestr(now,'yyyy');
      | else
      |     first = first(end-3:end);  %year is last four digits
      | end
      | 
      | last = get_param(sys,'LastModifiedDate');
      | if isempty(last)
      |     last = datestr(now,'yyyy');
      | else
      |     last = last(end-3:end);
      | end
      | 
      | if strcmp(first,last)
      |     fprintf('%s\nCopyright  %s Nexteer',NxtrConf,first);
      | else
      |     fprintf('%s\n%s%s-%s Nexteer',NxtrConf,char(169),first,last);
      | end
  Data Store Write : DataStoreWrite  DataStoreName=DutyCycExcddCntQlfr
  Data Store Write2 : DataStoreWrite  DataStoreName=DutyCycExcddCntStInfo
  Data Store Write3 : DataStoreWrite  DataStoreName=DutyCycExcddCntStsVal
  Data Type Conversion : DataTypeConversion  OutDataTypeStr=Enum: SigQlfr1
  Ground : Ground
  ISO Fault Debounce Design : Stateflow chart  TreatAsAtomicUnit=on
      settings: AttributesFormatString=|
      | Simulation Purpose Only.
      | Do Not Code this block
      | Diagnostic Manager Owns this requirement
  Terminator : Terminator
  Terminator1 : Terminator
  wires:
  Data Type Conversion/1 -> Data Store Write/1
  ISO Fault Debounce Design/1(Qualifier) -> Data Type Conversion/1
  NtcSts/1 -> Data Store Write3/1, ISO Fault Debounce Design/1(NtcSts)
  Ground/1 -> ISO Fault Debounce Design/3(SvcClr)
  DebStep/1 -> ISO Fault Debounce Design/2(DebStep)
  NtcStInfo/1 -> Terminator1/1, Data Store Write2/1
  NtcNr/1 -> Terminator/1

== system SF009A_DutyCycThermProtn/DutyCycThermProtn/DutyCycThermProtnPer1/ThermalLimitStatus/MaxoutLimiting/SetNtcPass/Copyright1 ==

== system SF009A_DutyCycThermProtn/DutyCycThermProtn/DutyCycThermProtnPer1/ThermalLimitStatus/MaxoutLimiting/SetNtcPass/SetNtcSts ==
  note: Note:
      |
      | - "ISO Fault Debounce Design" Simulink block intent to use here for Simulation purpose only. Do not Code this block
  NtcNr : Inport
  NtcStInfo : Inport  Port=2
  NtcSts : Inport  Port=3
  DebStep : Inport  Port=4
  Copyright1 : Subsystem  Description=|  RequirementInfo={} %GIDa_68ab169f_ef4f_4b38_90eb_a407b2cfc17b  mask(Copyright Information){none=on}
      | Copyright info block.                                               
      |                                                                     
      | Place copyright information at the top of every subsystem in design.
      mask prompts: none "No parameters"
      mask help: Place copyright information at the top of every subsystem in design.
      mask Display:
      | NxtrConf = 'Nexteer Confidential';
      | 
      | sys = bdroot; %handle for the current model ("system")
      | first = get_param(sys,'Created');
      | if(isempty(first))
      |     first = datestr(now,'yyyy');
      | else
      |     first = first(end-3:end);  %year is last four digits
      | end
      | 
      | last = get_param(sys,'LastModifiedDate');
      | if isempty(last)
      |     last = datestr(now,'yyyy');
      | else
      |     last = last(end-3:end);
      | end
      | 
      | if strcmp(first,last)
      |     fprintf('%s\nCopyright  %s Nexteer',NxtrConf,first);
      | else
      |     fprintf('%s\n%s%s-%s Nexteer',NxtrConf,char(169),first,last);
      | end
  Data Store Write : DataStoreWrite  DataStoreName=DutyCycExcddCntQlfr
  Data Store Write2 : DataStoreWrite  DataStoreName=DutyCycExcddCntStInfo
  Data Store Write3 : DataStoreWrite  DataStoreName=DutyCycExcddCntStsVal
  Data Type Conversion : DataTypeConversion  OutDataTypeStr=Enum: SigQlfr1
  Ground : Ground
  ISO Fault Debounce Design : Stateflow chart  TreatAsAtomicUnit=on
      settings: AttributesFormatString=|
      | Simulation Purpose Only.
      | Do Not Code this block
      | Diagnostic Manager Owns this requirement
  Terminator : Terminator
  Terminator1 : Terminator
  wires:
  Data Type Conversion/1 -> Data Store Write/1
  ISO Fault Debounce Design/1(Qualifier) -> Data Type Conversion/1
  NtcSts/1 -> Data Store Write3/1, ISO Fault Debounce Design/1(NtcSts)
  Ground/1 -> ISO Fault Debounce Design/3(SvcClr)
  DebStep/1 -> ISO Fault Debounce Design/2(DebStep)
  NtcStInfo/1 -> Terminator1/1, Data Store Write2/1
  NtcNr/1 -> Terminator/1

== system SF009A_DutyCycThermProtn/DutyCycThermProtn/DutyCycThermProtnPer1/ThermalLimitStatus/MaxoutLimiting/SetNtcFail/SetNtcSts/Copyright1 ==

== system SF009A_DutyCycThermProtn/DutyCycThermProtn/DutyCycThermProtnPer1/ThermalLimitStatus/MaxoutLimiting/SetNtcPass/SetNtcSts/Copyright1 ==
